simulink model "original"  (R2021b)
settings: Solver=VariableStepAuto  StartTime=0.0  StopTime=10.0  RelTol=1e-3
settings Model: Creator=user  LastModifiedBy=wangzixuan

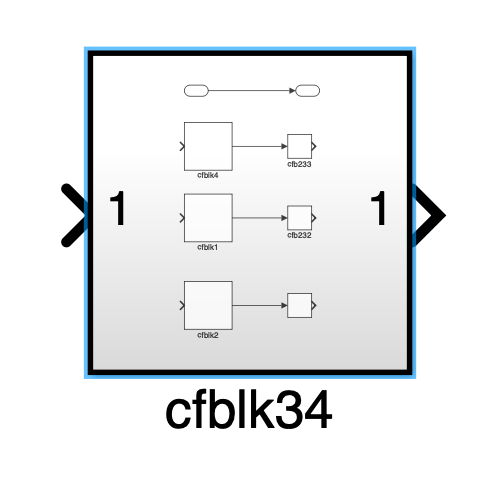
[thumbnail: Simulink's stored preview of the top-level diagram]
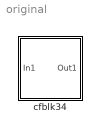
== system original ==
  cfblk34 : Subsystem  TreatAsAtomicUnit=on

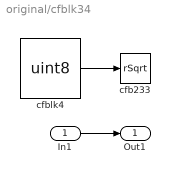
== system original/cfblk34 ==
  In1 : Inport
  cfb233 : Sqrt  Operator=rSqrt  SaturateOnIntegerOverflow=on
  cfblk4 : DataTypeConversion  OutDataTypeStr=uint8
  Out1 : Outport
  wires:
  In1/1 -> Out1/1
  cfblk4/1 -> cfb233/1
